simulink model "ppo_position_attitude4drone"  (R2025a)
settings: Solver=ode4  StartTime=0.0  StopTime=50  FixedStep=0.01  RelTol=1e-3
values from neighbouring files (symbols this model uses):
  control_noise = 0.045    [PPO_simulation.mat]    (also in TEST_POS_ATT_PPO.m)
  p_IC = IC(10)    [TEST_POS_ATT_PPO.m]
  phi_IC = IC(7)    [TEST_POS_ATT_PPO.m]
  psi_IC = IC(9)    [TEST_POS_ATT_PPO.m]
  q_IC = IC(11)    [TEST_POS_ATT_PPO.m]
  r_IC = IC(12)    [TEST_POS_ATT_PPO.m]
  state_noise = 0.045    [PPO_simulation.mat]    (also in TEST_POS_ATT_PPO.m)
  theta_IC = IC(8)    [TEST_POS_ATT_PPO.m]
  Ts_Sim = 0.01    [PPO_simulation.mat]    (also in TEST_POS_ATT_PPO.m)
  u_IC = IC(4)    [TEST_POS_ATT_PPO.m]
  v_IC = IC(5)    [TEST_POS_ATT_PPO.m]
  w_IC = IC(6)    [TEST_POS_ATT_PPO.m]
  x_IC = IC(1)    [TEST_POS_ATT_PPO.m]
  y_IC = IC(2)    [TEST_POS_ATT_PPO.m]
  z_IC = IC(3)    [TEST_POS_ATT_PPO.m]
undefined symbols (not defined in the file or in its folder): p_IC2, p_IC3, p_IC4, phi_IC2, phi_IC3, psi_IC2, psi_IC3, q_IC2, q_IC3, r_IC2, r_IC3, saturation_logic, theta_IC2, theta_IC3, u_IC2, u_IC3, v_IC2, v_IC3, w_IC2, w_IC3, wind_logic, x_IC2, x_IC3, y_IC2, y_IC3, z_IC2, z_IC3
libraries: rllib x8
(part 1 of 2)
settings Model: Creator=tn163528  LastModifiedBy=re606359

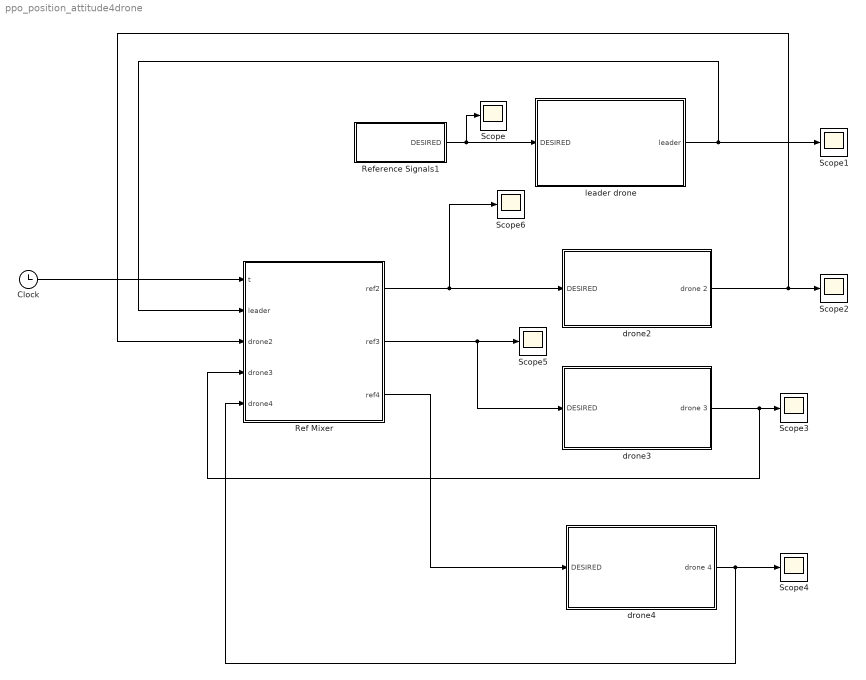
== system ppo_position_attitude4drone ==
  Clock : Clock
  Ref Mixer : MATLAB Function  TreatAsAtomicUnit=on
  Reference Signals1 : Subsystem
  Scope{,1..6} (7 alike) : Scope
      Scope settings: ActiveDisplayYMinimum=-18.329552788512615  ActiveDisplayYMaximum=13.709653230357763  DataLoggingVariableName=ScopeData4
      Scope1 settings: ActiveDisplayYMinimum=-16.8140847666006  ActiveDisplayYMaximum=12.7682316407334  DataLoggingVariableName=ScopeData5
      Scope2 settings: ActiveDisplayYMinimum=-6.2640011047441817  ActiveDisplayYMaximum=4.5374433382914088  DataLoggingVariableName=ScopeData6
      Scope3 settings: ActiveDisplayYMinimum=-16.848247513670785  ActiveDisplayYMaximum=11.660916390407865  DataLoggingVariableName=ScopeData7
      Scope4 settings: ActiveDisplayYMinimum=-16.848247513670785  ActiveDisplayYMaximum=11.660916390407865  DataLoggingVariableName=ScopeData8
      Scope5 settings: ActiveDisplayYMinimum=-2.7528365085187443  ActiveDisplayYMaximum=5.3529951795390245  DataLoggingVariableName=ScopeData9
      Scope6 settings: ActiveDisplayYMinimum=-18.051610011264458  ActiveDisplayYMaximum=3.5641646704603374  DataLoggingVariableName=ScopeData10
  drone2 : Subsystem
  drone3 : Subsystem
  drone4 : Subsystem
  leader drone : Subsystem
  wires:
  Clock/1 -> Ref Mixer/1(t)
  Reference Signals1/1(DESIRED) -> Scope/1, leader drone/1(DESIRED)
  leader drone/1(leader) -> Scope1/1, Ref Mixer/2(leader)
  drone2/1(drone 2) -> Ref Mixer/3(drone2), Scope2/1
  Ref Mixer/1(ref2) -> Scope6/1, drone2/1(DESIRED)
  Ref Mixer/2(ref3) -> drone3/1(DESIRED), Scope5/1
  drone3/1(drone 3) -> Ref Mixer/4(drone3), Scope3/1
  Ref Mixer/3(ref4) -> drone4/1(DESIRED)
  drone4/1(drone 4) -> Ref Mixer/5(drone4), Scope4/1

== system ppo_position_attitude4drone/Reference Signals1 ==
  Clock1 : Clock
  MATLAB Function : MATLAB Function  TreatAsAtomicUnit=on
  Mux : Mux  Inputs=6
  Mux1 : Mux  Inputs=6
  To Workspace : ToWorkspace  VariableName=X_ref  SampleTime=Ts_Sim
  DESIRED : Outport
  wires:
  MATLAB Function/5(z_desir) -> Mux1/3, Mux/5
  MATLAB Function/1(x_desir) -> Mux1/1, Mux/1
  MATLAB Function/6(z_d_desir) -> Mux1/6, Mux/6
  MATLAB Function/2(x_d_desir) -> Mux1/4, Mux/2
  MATLAB Function/3(y_desir) -> Mux1/2, Mux/3
  Mux/1 -> DESIRED/1
  MATLAB Function/4(y_d_desir) -> Mux1/5, Mux/4
  Mux1/1 -> To Workspace/1
  Clock1/1 -> MATLAB Function/1(t)

== system ppo_position_attitude4drone/drone2 ==
  DESIRED : Inport
  Clock : Clock
  Drone_Dynamic1 : Subsystem
  PPO_attitude_controller : Subsystem
  PPO_position_controller : Subsystem
  Scope : Scope  NumInputPorts=3
      settings: ActiveDisplayYMinimum=-0.22794541157782078  ActiveDisplayYMaximum=0.65998090244829655  DataLoggingVariableName=ScopeData2
  Scope1 : Scope
      settings: ActiveDisplayYMinimum=9.7400799288833344  ActiveDisplayYMaximum=10.440050935310733
  System_Solver : MATLAB Function  TreatAsAtomicUnit=on
  drone 2 : Outport
  wires:
  DESIRED/1 -> PPO_position_controller/1(DESIRED)
  PPO_position_controller/3(Uz) -> System_Solver/3(u_z)
  PPO_attitude_controller/1(Taux) -> Scope/3, Drone_Dynamic1/1(tau_x)
  Drone_Dynamic1/1(attitude) -> PPO_attitude_controller/1(actual)  "inner_loop"
  PPO_attitude_controller/2(Tauy) -> Scope/2, Drone_Dynamic1/2(tau_y)
  Drone_Dynamic1/2(position) -> drone 2/1, PPO_position_controller/2(ACTUAL)  "Outer_loop"
  PPO_position_controller/2(Uy) -> System_Solver/2(u_y)
  Clock/1 -> System_Solver/4(t)
  System_Solver/2(theta_desired) -> PPO_attitude_controller/3(theta_desired)
  PPO_attitude_controller/3(Tauz) -> Scope/1, Drone_Dynamic1/3(tau_z)
  System_Solver/1(phi_desired) -> PPO_attitude_controller/2(phi_desired)
  PPO_position_controller/1(Ux) -> System_Solver/1(u_x)
  System_Solver/3(psi_desired) -> PPO_attitude_controller/4(psi_desired)
  System_Solver/4(Ft_desired) -> Drone_Dynamic1/4(F_t), Scope1/1  "F_t"

== system ppo_position_attitude4drone/drone3 ==
  DESIRED : Inport
  Clock : Clock
  Drone_Dynamic1 : Subsystem
  PPO_attitude_controller : Subsystem
  PPO_position_controller : Subsystem
  Scope : Scope  NumInputPorts=3
      settings: ActiveDisplayYMinimum=-0.22794541157782078  ActiveDisplayYMaximum=0.65998090244829655  DataLoggingVariableName=ScopeData2
  Scope1 : Scope
      settings: ActiveDisplayYMinimum=9.7400799288833344  ActiveDisplayYMaximum=10.440050935310733
  System_Solver : MATLAB Function  TreatAsAtomicUnit=on
  drone 3 : Outport
  wires:
  System_Solver/4(Ft_desired) -> Scope1/1, Drone_Dynamic1/4(F_t)  "F_t"
  System_Solver/3(psi_desired) -> PPO_attitude_controller/4(psi_desired)
  PPO_position_controller/1(Ux) -> System_Solver/1(u_x)
  System_Solver/1(phi_desired) -> PPO_attitude_controller/2(phi_desired)
  PPO_attitude_controller/3(Tauz) -> Drone_Dynamic1/3(tau_z), Scope/1
  System_Solver/2(theta_desired) -> PPO_attitude_controller/3(theta_desired)
  Clock/1 -> System_Solver/4(t)
  PPO_position_controller/2(Uy) -> System_Solver/2(u_y)
  Drone_Dynamic1/2(position) -> drone 3/1, PPO_position_controller/2(ACTUAL)  "Outer_loop"
  PPO_attitude_controller/2(Tauy) -> Drone_Dynamic1/2(tau_y), Scope/2
  Drone_Dynamic1/1(attitude) -> PPO_attitude_controller/1(actual)  "inner_loop"
  PPO_attitude_controller/1(Taux) -> Drone_Dynamic1/1(tau_x), Scope/3
  PPO_position_controller/3(Uz) -> System_Solver/3(u_z)
  DESIRED/1 -> PPO_position_controller/1(DESIRED)

== system ppo_position_attitude4drone/drone4 ==
  DESIRED : Inport
  Clock : Clock
  Drone_Dynamic1 : Subsystem
  PPO_attitude_controller : Subsystem
  PPO_position_controller : Subsystem
  Scope : Scope  NumInputPorts=3
      settings: ActiveDisplayYMinimum=-0.22794541157782078  ActiveDisplayYMaximum=0.65998090244829655  DataLoggingVariableName=ScopeData2
  Scope1 : Scope
      settings: ActiveDisplayYMinimum=9.7400799288833344  ActiveDisplayYMaximum=10.440050935310733
  System_Solver : MATLAB Function  TreatAsAtomicUnit=on
  drone 4 : Outport
  wires:
  DESIRED/1 -> PPO_position_controller/1(DESIRED)
  PPO_position_controller/3(Uz) -> System_Solver/3(u_z)
  PPO_attitude_controller/1(Taux) -> Scope/3, Drone_Dynamic1/1(tau_x)
  Drone_Dynamic1/1(attitude) -> PPO_attitude_controller/1(actual)  "inner_loop"
  PPO_attitude_controller/2(Tauy) -> Scope/2, Drone_Dynamic1/2(tau_y)
  Drone_Dynamic1/2(position) -> PPO_position_controller/2(ACTUAL), drone 4/1  "Outer_loop"
  PPO_position_controller/2(Uy) -> System_Solver/2(u_y)
  Clock/1 -> System_Solver/4(t)
  System_Solver/2(theta_desired) -> PPO_attitude_controller/3(theta_desired)
  PPO_attitude_controller/3(Tauz) -> Scope/1, Drone_Dynamic1/3(tau_z)
  System_Solver/1(phi_desired) -> PPO_attitude_controller/2(phi_desired)
  PPO_position_controller/1(Ux) -> System_Solver/1(u_x)
  System_Solver/3(psi_desired) -> PPO_attitude_controller/4(psi_desired)
  System_Solver/4(Ft_desired) -> Drone_Dynamic1/4(F_t), Scope1/1  "F_t"

== system ppo_position_attitude4drone/leader drone ==
  DESIRED : Inport
  Clock : Clock
  Drone_Dynamic1 : Subsystem
  PPO_attitude_controller : Subsystem
  PPO_position_controller : Subsystem
  Scope : Scope  NumInputPorts=3
      settings: ActiveDisplayYMinimum=-0.26589944162275436  ActiveDisplayYMaximum=0.67670267800432526  DataLoggingVariableName=ScopeData12
  Scope1 : Scope
      settings: ActiveDisplayYMinimum=72.877153012049746  ActiveDisplayYMaximum=83.875579825299113  DataLoggingVariableName=ScopeData13
  System_Solver : MATLAB Function  TreatAsAtomicUnit=on
  leader : Outport
  wires:
  System_Solver/4(Ft_desired) -> Scope1/1, Drone_Dynamic1/4(F_t)  "F_t"
  PPO_attitude_controller/1(Taux) -> Drone_Dynamic1/1(tau_x), Scope/3
  System_Solver/1(phi_desired) -> PPO_attitude_controller/2(phi_desired)
  Clock/1 -> System_Solver/4(t)
  DESIRED/1 -> PPO_position_controller/1(DESIRED)
  PPO_position_controller/1(Ux) -> System_Solver/1(u_x)
  System_Solver/2(theta_desired) -> PPO_attitude_controller/3(theta_desired)
  Drone_Dynamic1/1(attitude) -> PPO_attitude_controller/1(actual)  "inner_loop"
  System_Solver/3(psi_desired) -> PPO_attitude_controller/4(psi_desired)
  PPO_position_controller/2(Uy) -> System_Solver/2(u_y)
  Drone_Dynamic1/2(position) -> leader/1, PPO_position_controller/2(ACTUAL)  "Outer_loop"
  PPO_position_controller/3(Uz) -> System_Solver/3(u_z)
  PPO_attitude_controller/2(Tauy) -> Drone_Dynamic1/2(tau_y), Scope/2
  PPO_attitude_controller/3(Tauz) -> Drone_Dynamic1/3(tau_z), Scope/1

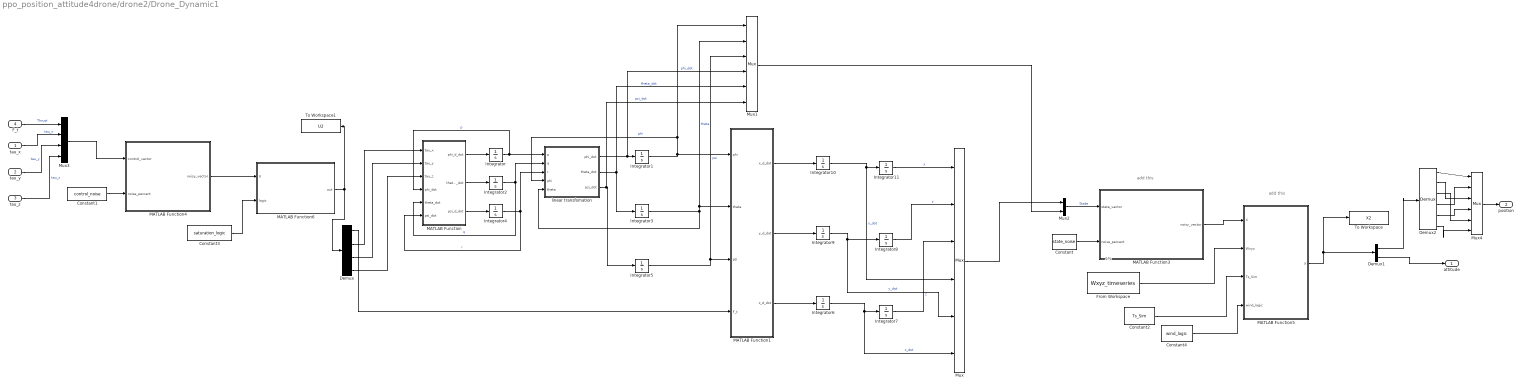
== system ppo_position_attitude4drone/drone2/Drone_Dynamic1 ==
  note: 1%
  note: add this
  note: add this
  tau_x : Inport
  tau_y : Inport  Port=2
  tau_z : Inport  Port=3
  F_t : Inport  Port=4
  Constant : Constant  Value=state_noise  SampleTime=Ts_Sim
  Constant1 : Constant  Value=control_noise
  Constant2 : Constant  Value=Ts_Sim
  Constant3 : Constant  Value=saturation_logic  SampleTime=Ts_Sim
  Constant4 : Constant  Value=wind_logic
  Demux : Demux
  Demux1 : Demux  Outputs=2
  Demux2 : Demux  Outputs=6
  From Workspace : FromWorkspace  VariableName=Wxyz_timeseries  SampleTime=Ts_Sim
  Integrator : Integrator  InitialCondition=p_IC2
  Integrator1 : Integrator  InitialCondition=phi_IC2
  Integrator10 : Integrator  InitialCondition=u_IC2
  Integrator11 : Integrator  InitialCondition=x_IC2
  Integrator2 : Integrator  InitialCondition=q_IC2
  Integrator3 : Integrator  InitialCondition=theta_IC2
  Integrator4 : Integrator  InitialCondition=r_IC2
  Integrator5 : Integrator  InitialCondition=psi_IC2
  Integrator6 : Integrator  InitialCondition=w_IC2
  Integrator7 : Integrator  InitialCondition=z_IC2
  Integrator8 : Integrator  InitialCondition=y_IC2
  Integrator9 : Integrator  InitialCondition=v_IC2
  MATLAB Function : MATLAB Function  TreatAsAtomicUnit=on
  MATLAB Function1 : MATLAB Function  TreatAsAtomicUnit=on
  MATLAB Function3 : MATLAB Function  TreatAsAtomicUnit=on
  MATLAB Function4 : MATLAB Function  TreatAsAtomicUnit=on
  MATLAB Function5 : MATLAB Function  TreatAsAtomicUnit=on
  MATLAB Function6 : MATLAB Function  TreatAsAtomicUnit=on
  Mux : Mux  Inputs=6
  Mux1 : Mux  Inputs=6
  Mux2 : Mux  Inputs=2
  Mux3 : Mux
  Mux4 : Mux  Inputs=6
  To Workspace : ToWorkspace  VariableName=X2  SampleTime=Ts_Sim
  To Workspace1 : ToWorkspace  VariableName=U2  SampleTime=Ts_Sim
  linear transfomation : MATLAB Function  TreatAsAtomicUnit=on
  attitude : Outport
  position : Outport  Port=2
  wires:
  Constant4/1 -> MATLAB Function5/4(wind_logic)
  Mux4/1 -> position/1
  Demux2/6 -> Mux4/6
  Demux2/3 -> Mux4/5
  Demux2/5 -> Mux4/4
  Demux2/2 -> Mux4/3
  Demux2/4 -> Mux4/2
  Demux2/1 -> Mux4/1
  Demux1/1 -> Demux2/1
  Integrator7/1 -> Mux/3  "z"
  Integrator8/1 -> Mux/2  "y"
  Demux/4 -> MATLAB Function/3(tau_z)
  Demux/3 -> MATLAB Function/2(tau_y)
  Demux/2 -> MATLAB Function/1(tau_x)
  Demux/1 -> MATLAB Function1/4(F_t)
  Mux3/1 -> MATLAB Function4/1(control_vector)
  tau_z/1 -> Mux3/4  "tau_z"
  tau_y/1 -> Mux3/3  "tau_y"
  tau_x/1 -> Mux3/2  "tau_x"
  F_t/1 -> Mux3/1  "Thrust"
  Constant1/1 -> MATLAB Function4/2(noise_percent)
  MATLAB Function6/1(out) -> To Workspace1/1, Demux/1
  Constant3/1 -> MATLAB Function6/2(logic)
  MATLAB Function4/1(noisy_vector) -> MATLAB Function6/1(U)
  Mux1/1 -> Mux2/2
  Mux/1 -> Mux2/1
  MATLAB Function5/1(X) -> Demux1/1, To Workspace/1
  Constant2/1 -> MATLAB Function5/3(Ts_Sim)
  From Workspace/1 -> MATLAB Function5/2(Wxyz)
  Demux1/2 -> attitude/1
  MATLAB Function3/1(noisy_vector) -> MATLAB Function5/1("X ")
  Constant/1 -> MATLAB Function3/2(noise_percent)
  Mux2/1 -> MATLAB Function3/1(state_vector)  "State"
  Integrator11/1 -> Mux/1  "x"
  linear transfomation/3(psi_dot) -> Integrator5/1, Mux1/6  "psi_dot"
  linear transfomation/2(theta_dot) -> Integrator3/1, Mux1/5  "theta_dot"
  linear transfomation/1(phi_dot) -> Integrator1/1, Mux1/4  "phi_dot"
  MATLAB Function/2(theta_d_dot) -> Integrator2/1
  MATLAB Function/1(phi_d_dot) -> Integrator/1
  MATLAB Function/3(psi_d_dot) -> Integrator4/1
  Integrator/1 -> linear transfomation/1(p), MATLAB Function/4(phi_dot)  "p"
  Integrator4/1 -> linear transfomation/3(r), MATLAB Function/6(psi_dot)  "r"
  Integrator2/1 -> linear transfomation/2(q), MATLAB Function/5(theta_dot)  "q"
  Integrator6/1 -> Integrator7/1, Mux/6  "z_dot"
  Integrator9/1 -> Integrator8/1, Mux/5  "y_dot"
  Integrator10/1 -> Integrator11/1, Mux/4  "x_dot"
  Integrator5/1 -> MATLAB Function1/3(psi), Mux1/3  "psi"
  Integrator3/1 -> linear transfomation/5(theta), MATLAB Function1/2(theta), Mux1/2  "theta"
  Integrator1/1 -> MATLAB Function1/1(phi), linear transfomation/4(phi), Mux1/1  "phi"
  MATLAB Function1/3(z_d_dot) -> Integrator6/1
  MATLAB Function1/2(y_d_dot) -> Integrator9/1
  MATLAB Function1/1(x_d_dot) -> Integrator10/1

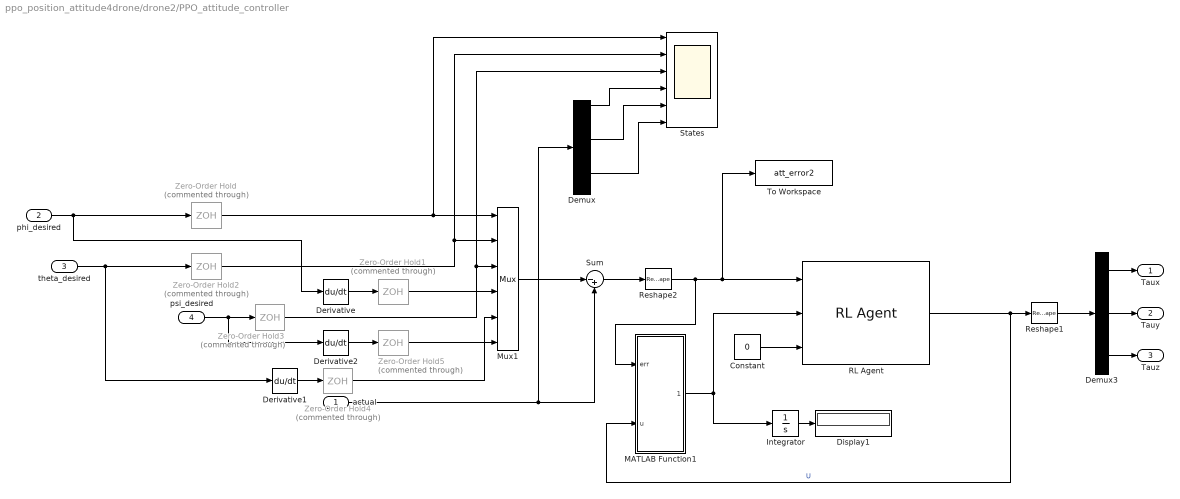
== system ppo_position_attitude4drone/drone2/PPO_attitude_controller ==
  actual : Inport
  phi_desired : Inport  Port=2
  theta_desired : Inport  Port=3
  psi_desired : Inport  Port=4
  Constant : Constant  Value=0
  Demux : Demux  Outputs=6
  Demux3 : Demux  Outputs=3
  Derivative : Derivative
  Derivative1 : Derivative
  Derivative2 : Derivative
  Display1 : Display
  Integrator : Integrator
  MATLAB Function1 : MATLAB Function  TreatAsAtomicUnit=on
  Mux1 : Mux  Inputs=6
  RL Agent : rllib/RL Agent  Agent=agent1  ExternalActionAsInput=off  ProvideLastAction=off  ProvideCumRwd=off  TreatAsDirectFeedthrough=on  UseStrictObservationDataTypes=off
  Reshape1 : Reshape
  Reshape2 : Reshape  OutputDimensionality=Column vector (2-D)
  States : Scope  NumInputPorts=6
      settings: ActiveDisplayYMinimum=-0.042848507934818772  ActiveDisplayYMaximum=0.10576663107375736
  Sum : Sum  Inputs=|-+
  To Workspace : ToWorkspace  VariableName=att_error2  SampleTime=Ts_Sim
  Zero-Order Hold{,1..5} (6 alike) : ZeroOrderHold  Commented=through  SampleTime=.1
  Taux : Outport
  Tauy : Outport  Port=2
  Tauz : Outport  Port=3
  wires:
  Zero-Order Hold5/1 -> Mux1/6
  Zero-Order Hold4/1 -> Mux1/5
  Zero-Order Hold3/1 -> Mux1/3, States/3
  Zero-Order Hold2/1 -> States/2, Mux1/2
  Zero-Order Hold1/1 -> Mux1/4
  Zero-Order Hold/1 -> States/1, Mux1/1
  Derivative2/1 -> Zero-Order Hold5/1
  Derivative1/1 -> Zero-Order Hold4/1
  Derivative/1 -> Zero-Order Hold1/1
  Demux/5 -> States/6
  Demux/3 -> States/5
  Demux/1 -> States/4
  Integrator/1 -> Display1/1
  MATLAB Function1/1(reward) -> Integrator/1, RL Agent/2
  Reshape2/1 -> MATLAB Function1/1(err), RL Agent/1, To Workspace/1
  Sum/1 -> Reshape2/1
  actual/1 -> Sum/2, Demux/1
  Mux1/1 -> Sum/1
  Reshape1/1 -> Demux3/1
  psi_desired/1 -> Zero-Order Hold3/1, Derivative2/1
  theta_desired/1 -> Derivative1/1, Zero-Order Hold2/1
  phi_desired/1 -> Derivative/1, Zero-Order Hold/1
  Demux3/3 -> Tauz/1
  Demux3/2 -> Tauy/1
  Demux3/1 -> Taux/1
  Constant/1 -> RL Agent/3
  RL Agent/1 -> Reshape1/1, MATLAB Function1/2(u)  "U"

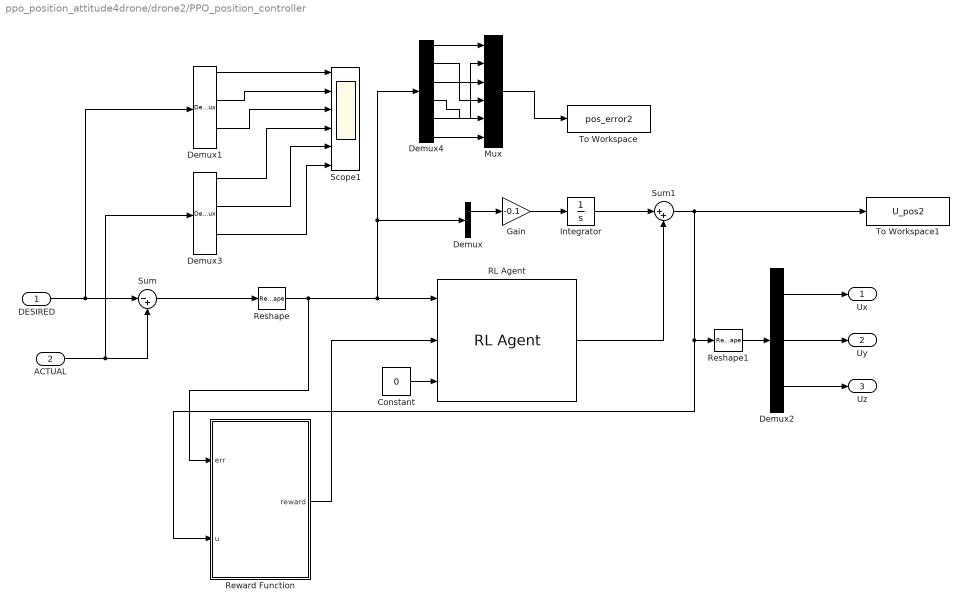
== system ppo_position_attitude4drone/drone2/PPO_position_controller ==
  DESIRED : Inport
  ACTUAL : Inport  Port=2
  Constant : Constant  Value=0
  Demux : Demux  Outputs=2
  Demux1 : Demux  Outputs=6
  Demux2 : Demux  Outputs=3
  Demux3 : Demux  Outputs=6
  Demux4 : Demux  Outputs=6
  Gain : Gain  Gain=-0.1
  Integrator : Integrator
  Mux : Mux  Inputs=6
  RL Agent : rllib/RL Agent  Agent=agent  ExternalActionAsInput=off  ProvideLastAction=off  ProvideCumRwd=off  TreatAsDirectFeedthrough=on  UseStrictObservationDataTypes=off
  Reshape : Reshape  OutputDimensionality=Column vector (2-D)
  Reshape1 : Reshape
  Reward Function : MATLAB Function  TreatAsAtomicUnit=on
  Scope1 : Scope  NumInputPorts=6
      settings: ActiveDisplayYMinimum=-5.046617163465049  ActiveDisplayYMaximum=4.1195544711854284
  Sum : Sum  Inputs=|-+
  Sum1 : Sum  Inputs=|++
  To Workspace : ToWorkspace  VariableName=pos_error2  SampleTime=Ts_Sim
  To Workspace1 : ToWorkspace  VariableName=U_pos2  SampleTime=Ts_Sim
  Ux : Outport
  Uy : Outport  Port=2
  Uz : Outport  Port=3
  wires:
  RL Agent/1 -> Sum1/2
  Demux4/6 -> Mux/6
  Demux4/4 -> Mux/5
  Demux4/5 -> Mux/3
  Demux4/3 -> Mux/2
  Demux4/2 -> Mux/4
  Mux/1 -> To Workspace/1
  Demux4/1 -> Mux/1
  Sum1/1 -> Reshape1/1, Reward Function/2(u), To Workspace1/1
  Integrator/1 -> Sum1/1
  Demux/1 -> Gain/1
  Gain/1 -> Integrator/1
  Demux3/5 -> Scope1/6
  Demux3/3 -> Scope1/5
  Demux3/1 -> Scope1/4
  Demux1/5 -> Scope1/3
  Demux1/3 -> Scope1/2
  Demux1/1 -> Scope1/1
  Constant/1 -> RL Agent/3
  Reshape/1 -> Reward Function/1(err), RL Agent/1, Demux4/1, Demux/1
  Sum/1 -> Reshape/1
  DESIRED/1 -> Sum/1, Demux1/1
  ACTUAL/1 -> Sum/2, Demux3/1
  Reward Function/1(reward) -> RL Agent/2
  Reshape1/1 -> Demux2/1
  Demux2/3 -> Uz/1
  Demux2/2 -> Uy/1
  Demux2/1 -> Ux/1

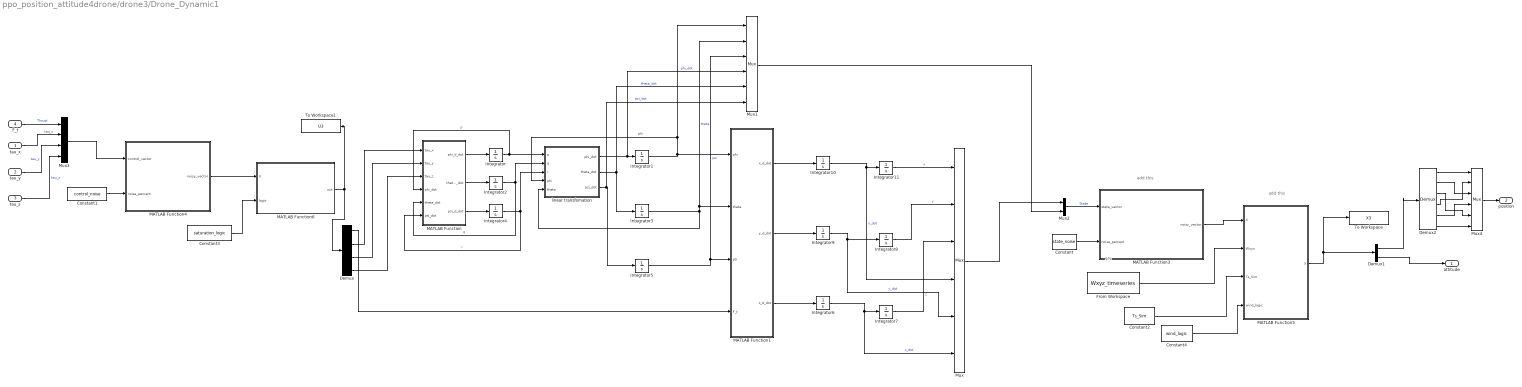
== system ppo_position_attitude4drone/drone3/Drone_Dynamic1 ==
  note: add this
  note: add this
  note: 1%
  tau_x : Inport
  tau_y : Inport  Port=2
  tau_z : Inport  Port=3
  F_t : Inport  Port=4
  Constant : Constant  Value=state_noise  SampleTime=Ts_Sim
  Constant1 : Constant  Value=control_noise
  Constant2 : Constant  Value=Ts_Sim
  Constant3 : Constant  Value=saturation_logic  SampleTime=Ts_Sim
  Constant4 : Constant  Value=wind_logic
  Demux : Demux
  Demux1 : Demux  Outputs=2
  Demux2 : Demux  Outputs=6
  From Workspace : FromWorkspace  VariableName=Wxyz_timeseries  SampleTime=Ts_Sim
  Integrator : Integrator  InitialCondition=p_IC3
  Integrator1 : Integrator  InitialCondition=phi_IC3
  Integrator10 : Integrator  InitialCondition=u_IC3
  Integrator11 : Integrator  InitialCondition=x_IC3
  Integrator2 : Integrator  InitialCondition=q_IC3
  Integrator3 : Integrator  InitialCondition=theta_IC3
  Integrator4 : Integrator  InitialCondition=r_IC3
  Integrator5 : Integrator  InitialCondition=psi_IC3
  Integrator6 : Integrator  InitialCondition=w_IC3
  Integrator7 : Integrator  InitialCondition=z_IC3
  Integrator8 : Integrator  InitialCondition=y_IC3
  Integrator9 : Integrator  InitialCondition=v_IC3
  MATLAB Function : MATLAB Function  TreatAsAtomicUnit=on
  MATLAB Function1 : MATLAB Function  TreatAsAtomicUnit=on
  MATLAB Function3 : MATLAB Function  TreatAsAtomicUnit=on
  MATLAB Function4 : MATLAB Function  TreatAsAtomicUnit=on
  MATLAB Function5 : MATLAB Function  TreatAsAtomicUnit=on
  MATLAB Function6 : MATLAB Function  TreatAsAtomicUnit=on
  Mux : Mux  Inputs=6
  Mux1 : Mux  Inputs=6
  Mux2 : Mux  Inputs=2
  Mux3 : Mux
  Mux4 : Mux  Inputs=6
  To Workspace : ToWorkspace  VariableName=X3  SampleTime=Ts_Sim
  To Workspace1 : ToWorkspace  VariableName=U3  SampleTime=Ts_Sim
  linear transfomation : MATLAB Function  TreatAsAtomicUnit=on
  attitude : Outport
  position : Outport  Port=2
  wires:
  MATLAB Function1/1(x_d_dot) -> Integrator10/1
  MATLAB Function1/2(y_d_dot) -> Integrator9/1
  MATLAB Function1/3(z_d_dot) -> Integrator6/1
  Integrator1/1 -> Mux1/1, linear transfomation/4(phi), MATLAB Function1/1(phi)  "phi"
  Integrator3/1 -> Mux1/2, MATLAB Function1/2(theta), linear transfomation/5(theta)  "theta"
  Integrator5/1 -> Mux1/3, MATLAB Function1/3(psi)  "psi"
  Integrator10/1 -> Mux/4, Integrator11/1  "x_dot"
  Integrator9/1 -> Mux/5, Integrator8/1  "y_dot"
  Integrator6/1 -> Mux/6, Integrator7/1  "z_dot"
  Integrator2/1 -> MATLAB Function/5(theta_dot), linear transfomation/2(q)  "q"
  Integrator4/1 -> MATLAB Function/6(psi_dot), linear transfomation/3(r)  "r"
  Integrator/1 -> MATLAB Function/4(phi_dot), linear transfomation/1(p)  "p"
  MATLAB Function/3(psi_d_dot) -> Integrator4/1
  MATLAB Function/1(phi_d_dot) -> Integrator/1
  MATLAB Function/2(theta_d_dot) -> Integrator2/1
  linear transfomation/1(phi_dot) -> Mux1/4, Integrator1/1  "phi_dot"
  linear transfomation/2(theta_dot) -> Mux1/5, Integrator3/1  "theta_dot"
  linear transfomation/3(psi_dot) -> Mux1/6, Integrator5/1  "psi_dot"
  Integrator11/1 -> Mux/1  "x"
  Mux2/1 -> MATLAB Function3/1(state_vector)  "State"
  Constant/1 -> MATLAB Function3/2(noise_percent)
  MATLAB Function3/1(noisy_vector) -> MATLAB Function5/1("X ")
  Demux1/2 -> attitude/1
  From Workspace/1 -> MATLAB Function5/2(Wxyz)
  Constant2/1 -> MATLAB Function5/3(Ts_Sim)
  MATLAB Function5/1(X) -> To Workspace/1, Demux1/1
  Mux/1 -> Mux2/1
  Mux1/1 -> Mux2/2
  MATLAB Function4/1(noisy_vector) -> MATLAB Function6/1(U)
  Constant3/1 -> MATLAB Function6/2(logic)
  MATLAB Function6/1(out) -> Demux/1, To Workspace1/1
  Constant1/1 -> MATLAB Function4/2(noise_percent)
  F_t/1 -> Mux3/1  "Thrust"
  tau_x/1 -> Mux3/2  "tau_x"
  tau_y/1 -> Mux3/3  "tau_y"
  tau_z/1 -> Mux3/4  "tau_z"
  Mux3/1 -> MATLAB Function4/1(control_vector)
  Demux/1 -> MATLAB Function1/4(F_t)
  Demux/2 -> MATLAB Function/1(tau_x)
  Demux/3 -> MATLAB Function/2(tau_y)
  Demux/4 -> MATLAB Function/3(tau_z)
  Integrator8/1 -> Mux/2  "y"
  Integrator7/1 -> Mux/3  "z"
  Demux1/1 -> Demux2/1
  Demux2/1 -> Mux4/1
  Demux2/4 -> Mux4/2
  Demux2/2 -> Mux4/3
  Demux2/5 -> Mux4/4
  Demux2/3 -> Mux4/5
  Demux2/6 -> Mux4/6
  Mux4/1 -> position/1
  Constant4/1 -> MATLAB Function5/4(wind_logic)

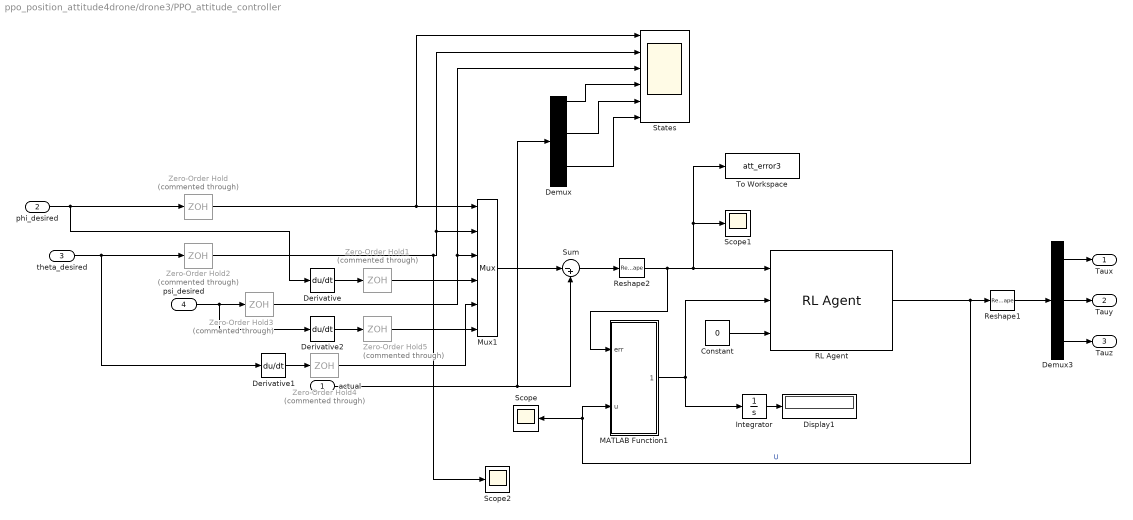
== system ppo_position_attitude4drone/drone3/PPO_attitude_controller ==
  actual : Inport
  phi_desired : Inport  Port=2
  theta_desired : Inport  Port=3
  psi_desired : Inport  Port=4
  Constant : Constant  Value=0
  Demux : Demux  Outputs=6
  Demux3 : Demux  Outputs=3
  Derivative : Derivative
  Derivative1 : Derivative
  Derivative2 : Derivative
  Display1 : Display
  Integrator : Integrator
  MATLAB Function1 : MATLAB Function  TreatAsAtomicUnit=on
  Mux1 : Mux  Inputs=6
  RL Agent : rllib/RL Agent  Agent=agent1  ExternalActionAsInput=off  ProvideLastAction=off  ProvideCumRwd=off  TreatAsDirectFeedthrough=on  UseStrictObservationDataTypes=off
  Reshape1 : Reshape
  Reshape2 : Reshape  OutputDimensionality=Column vector (2-D)
  Scope : Scope
      settings: ActiveDisplayYMinimum=-0.20127  ActiveDisplayYMaximum=0.69251
  Scope1 : Scope
      settings: ActiveDisplayYMinimum=-1  ActiveDisplayYMaximum=1
  Scope2 : Scope
      settings: ActiveDisplayYMinimum=-0.040406254965963853  ActiveDisplayYMaximum=0.036209580605539526  DataLoggingVariableName=ScopeData3
  States : Scope  NumInputPorts=6
      settings: ActiveDisplayYMinimum=-0.042848507934818772  ActiveDisplayYMaximum=0.10576663107375736
  Sum : Sum  Inputs=|-+
  To Workspace : ToWorkspace  VariableName=att_error3  SampleTime=Ts_Sim
  Zero-Order Hold{,1..5} (6 alike) : ZeroOrderHold  Commented=through  SampleTime=.1
  Taux : Outport
  Tauy : Outport  Port=2
  Tauz : Outport  Port=3
  wires:
  RL Agent/1 -> Scope/1, MATLAB Function1/2(u), Reshape1/1  "U"
  Constant/1 -> RL Agent/3
  Demux3/1 -> Taux/1
  Demux3/2 -> Tauy/1
  Demux3/3 -> Tauz/1
  phi_desired/1 -> Zero-Order Hold/1, Derivative/1
  theta_desired/1 -> Zero-Order Hold2/1, Derivative1/1
  psi_desired/1 -> Derivative2/1, Zero-Order Hold3/1
  Reshape1/1 -> Demux3/1
  Mux1/1 -> Sum/1
  actual/1 -> Demux/1, Sum/2
  Sum/1 -> Reshape2/1
  Reshape2/1 -> To Workspace/1, Scope1/1, RL Agent/1, MATLAB Function1/1(err)
  MATLAB Function1/1(reward) -> RL Agent/2, Integrator/1
  Integrator/1 -> Display1/1
  Demux/1 -> States/4
  Demux/3 -> States/5
  Demux/5 -> States/6
  Derivative/1 -> Zero-Order Hold1/1
  Derivative1/1 -> Zero-Order Hold4/1
  Derivative2/1 -> Zero-Order Hold5/1
  Zero-Order Hold/1 -> Mux1/1, States/1
  Zero-Order Hold1/1 -> Mux1/4
  Zero-Order Hold2/1 -> Scope2/1, Mux1/2, States/2
  Zero-Order Hold3/1 -> States/3, Mux1/3
  Zero-Order Hold4/1 -> Mux1/5
  Zero-Order Hold5/1 -> Mux1/6

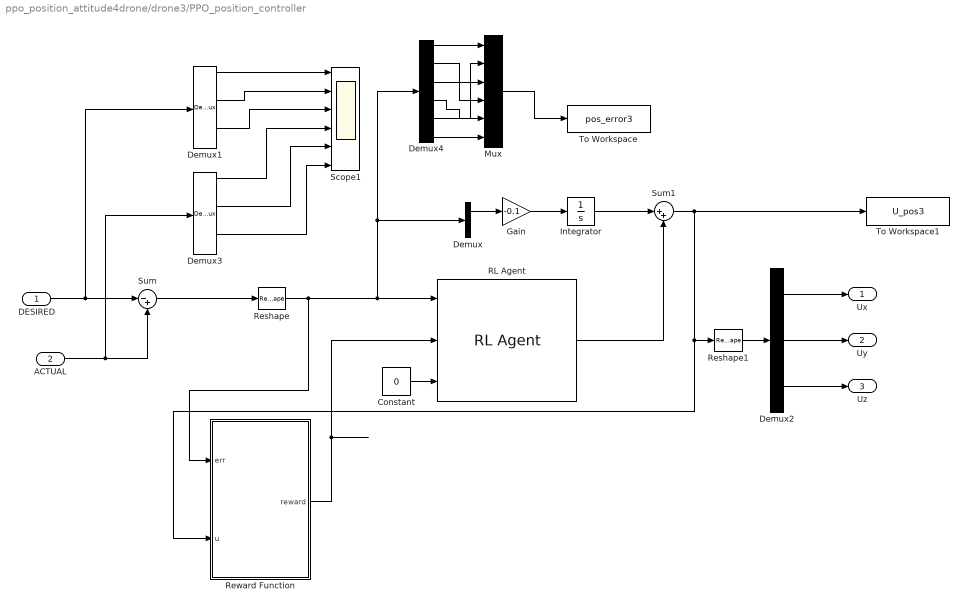
== system ppo_position_attitude4drone/drone3/PPO_position_controller ==
  DESIRED : Inport
  ACTUAL : Inport  Port=2
  Constant : Constant  Value=0
  Demux : Demux  Outputs=2
  Demux1 : Demux  Outputs=6
  Demux2 : Demux  Outputs=3
  Demux3 : Demux  Outputs=6
  Demux4 : Demux  Outputs=6
  Gain : Gain  Gain=-0.1
  Integrator : Integrator
  Mux : Mux  Inputs=6
  RL Agent : rllib/RL Agent  Agent=agent  ExternalActionAsInput=off  ProvideLastAction=off  ProvideCumRwd=off  TreatAsDirectFeedthrough=on  UseStrictObservationDataTypes=off
  Reshape : Reshape  OutputDimensionality=Column vector (2-D)
  Reshape1 : Reshape
  Reward Function : MATLAB Function  TreatAsAtomicUnit=on
  Scope1 : Scope  NumInputPorts=6
      settings: ActiveDisplayYMinimum=-5.046617163465049  ActiveDisplayYMaximum=4.1195544711854284
  Sum : Sum  Inputs=|-+
  Sum1 : Sum  Inputs=|++
  To Workspace : ToWorkspace  VariableName=pos_error3  SampleTime=Ts_Sim
  To Workspace1 : ToWorkspace  VariableName=U_pos3  SampleTime=Ts_Sim
  Ux : Outport
  Uy : Outport  Port=2
  Uz : Outport  Port=3
  wires:
  Demux2/1 -> Ux/1
  Demux2/2 -> Uy/1
  Demux2/3 -> Uz/1
  Reshape1/1 -> Demux2/1
  Reward Function/1(reward) -> RL Agent/2
  ACTUAL/1 -> Demux3/1, Sum/2
  DESIRED/1 -> Demux1/1, Sum/1
  Sum/1 -> Reshape/1
  Reshape/1 -> Demux/1, Demux4/1, RL Agent/1, Reward Function/1(err)
  Constant/1 -> RL Agent/3
  Demux1/1 -> Scope1/1
  Demux1/3 -> Scope1/2
  Demux1/5 -> Scope1/3
  Demux3/1 -> Scope1/4
  Demux3/3 -> Scope1/5
  Demux3/5 -> Scope1/6
  Gain/1 -> Integrator/1
  Demux/1 -> Gain/1
  Integrator/1 -> Sum1/1
  Sum1/1 -> To Workspace1/1, Reward Function/2(u), Reshape1/1
  Demux4/1 -> Mux/1
  Mux/1 -> To Workspace/1
  Demux4/2 -> Mux/4
  Demux4/3 -> Mux/2
  Demux4/5 -> Mux/3
  Demux4/4 -> Mux/5
  Demux4/6 -> Mux/6
  RL Agent/1 -> Sum1/2

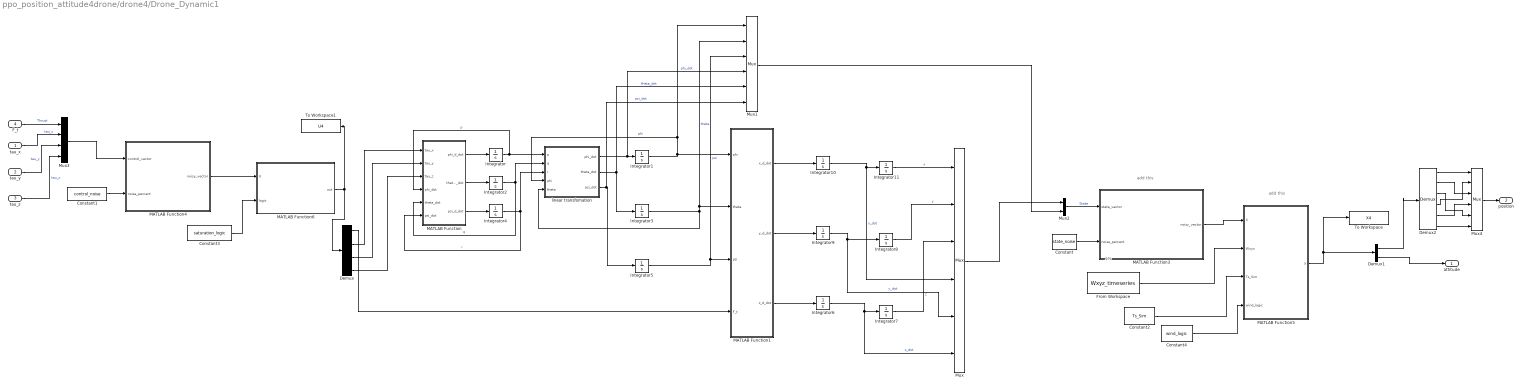
== system ppo_position_attitude4drone/drone4/Drone_Dynamic1 ==
  note: 1%
  note: add this
  note: add this
  tau_x : Inport
  tau_y : Inport  Port=2
  tau_z : Inport  Port=3
  F_t : Inport  Port=4
  Constant : Constant  Value=state_noise  SampleTime=Ts_Sim
  Constant1 : Constant  Value=control_noise
  Constant2 : Constant  Value=Ts_Sim
  Constant3 : Constant  Value=saturation_logic  SampleTime=Ts_Sim
  Constant4 : Constant  Value=wind_logic
  Demux : Demux
  Demux1 : Demux  Outputs=2
  Demux2 : Demux  Outputs=6
  From Workspace : FromWorkspace  VariableName=Wxyz_timeseries  SampleTime=Ts_Sim
  Integrator : Integrator  InitialCondition=p_IC4
  Integrator1 : Integrator  InitialCondition=phi_IC3
  Integrator10 : Integrator  InitialCondition=u_IC3
  Integrator11 : Integrator  InitialCondition=x_IC3
  Integrator2 : Integrator  InitialCondition=q_IC3
  Integrator3 : Integrator  InitialCondition=theta_IC3
  Integrator4 : Integrator  InitialCondition=r_IC3
  Integrator5 : Integrator  InitialCondition=psi_IC3
  Integrator6 : Integrator  InitialCondition=w_IC3
  Integrator7 : Integrator  InitialCondition=z_IC3
  Integrator8 : Integrator  InitialCondition=y_IC3
  Integrator9 : Integrator  InitialCondition=v_IC3
  MATLAB Function : MATLAB Function  TreatAsAtomicUnit=on
  MATLAB Function1 : MATLAB Function  TreatAsAtomicUnit=on
  MATLAB Function3 : MATLAB Function  TreatAsAtomicUnit=on
  MATLAB Function4 : MATLAB Function  TreatAsAtomicUnit=on
  MATLAB Function5 : MATLAB Function  TreatAsAtomicUnit=on
  MATLAB Function6 : MATLAB Function  TreatAsAtomicUnit=on
  Mux : Mux  Inputs=6
  Mux1 : Mux  Inputs=6
  Mux2 : Mux  Inputs=2
  Mux3 : Mux
  Mux4 : Mux  Inputs=6
  To Workspace : ToWorkspace  VariableName=X4  SampleTime=Ts_Sim
  To Workspace1 : ToWorkspace  VariableName=U4  SampleTime=Ts_Sim
  linear transfomation : MATLAB Function  TreatAsAtomicUnit=on
  attitude : Outport
  position : Outport  Port=2
  wires:
  Constant4/1 -> MATLAB Function5/4(wind_logic)
  Mux4/1 -> position/1
  Demux2/6 -> Mux4/6
  Demux2/3 -> Mux4/5
  Demux2/5 -> Mux4/4
  Demux2/2 -> Mux4/3
  Demux2/4 -> Mux4/2
  Demux2/1 -> Mux4/1
  Demux1/1 -> Demux2/1
  Integrator7/1 -> Mux/3  "z"
  Integrator8/1 -> Mux/2  "y"
  Demux/4 -> MATLAB Function/3(tau_z)
  Demux/3 -> MATLAB Function/2(tau_y)
  Demux/2 -> MATLAB Function/1(tau_x)
  Demux/1 -> MATLAB Function1/4(F_t)
  Mux3/1 -> MATLAB Function4/1(control_vector)
  tau_z/1 -> Mux3/4  "tau_z"
  tau_y/1 -> Mux3/3  "tau_y"
  tau_x/1 -> Mux3/2  "tau_x"
  F_t/1 -> Mux3/1  "Thrust"
  Constant1/1 -> MATLAB Function4/2(noise_percent)
  MATLAB Function6/1(out) -> To Workspace1/1, Demux/1
  Constant3/1 -> MATLAB Function6/2(logic)
  MATLAB Function4/1(noisy_vector) -> MATLAB Function6/1(U)
  Mux1/1 -> Mux2/2
  Mux/1 -> Mux2/1
  MATLAB Function5/1(X) -> Demux1/1, To Workspace/1
  Constant2/1 -> MATLAB Function5/3(Ts_Sim)
  From Workspace/1 -> MATLAB Function5/2(Wxyz)
  Demux1/2 -> attitude/1
  MATLAB Function3/1(noisy_vector) -> MATLAB Function5/1("X ")
  Constant/1 -> MATLAB Function3/2(noise_percent)
  Mux2/1 -> MATLAB Function3/1(state_vector)  "State"
  Integrator11/1 -> Mux/1  "x"
  linear transfomation/3(psi_dot) -> Integrator5/1, Mux1/6  "psi_dot"
  linear transfomation/2(theta_dot) -> Integrator3/1, Mux1/5  "theta_dot"
  linear transfomation/1(phi_dot) -> Integrator1/1, Mux1/4  "phi_dot"
  MATLAB Function/2(theta_d_dot) -> Integrator2/1
  MATLAB Function/1(phi_d_dot) -> Integrator/1
  MATLAB Function/3(psi_d_dot) -> Integrator4/1
  Integrator/1 -> linear transfomation/1(p), MATLAB Function/4(phi_dot)  "p"
  Integrator4/1 -> linear transfomation/3(r), MATLAB Function/6(psi_dot)  "r"
  Integrator2/1 -> linear transfomation/2(q), MATLAB Function/5(theta_dot)  "q"
  Integrator6/1 -> Integrator7/1, Mux/6  "z_dot"
  Integrator9/1 -> Integrator8/1, Mux/5  "y_dot"
  Integrator10/1 -> Integrator11/1, Mux/4  "x_dot"
  Integrator5/1 -> MATLAB Function1/3(psi), Mux1/3  "psi"
  Integrator3/1 -> linear transfomation/5(theta), MATLAB Function1/2(theta), Mux1/2  "theta"
  Integrator1/1 -> MATLAB Function1/1(phi), linear transfomation/4(phi), Mux1/1  "phi"
  MATLAB Function1/3(z_d_dot) -> Integrator6/1
  MATLAB Function1/2(y_d_dot) -> Integrator9/1
  MATLAB Function1/1(x_d_dot) -> Integrator10/1

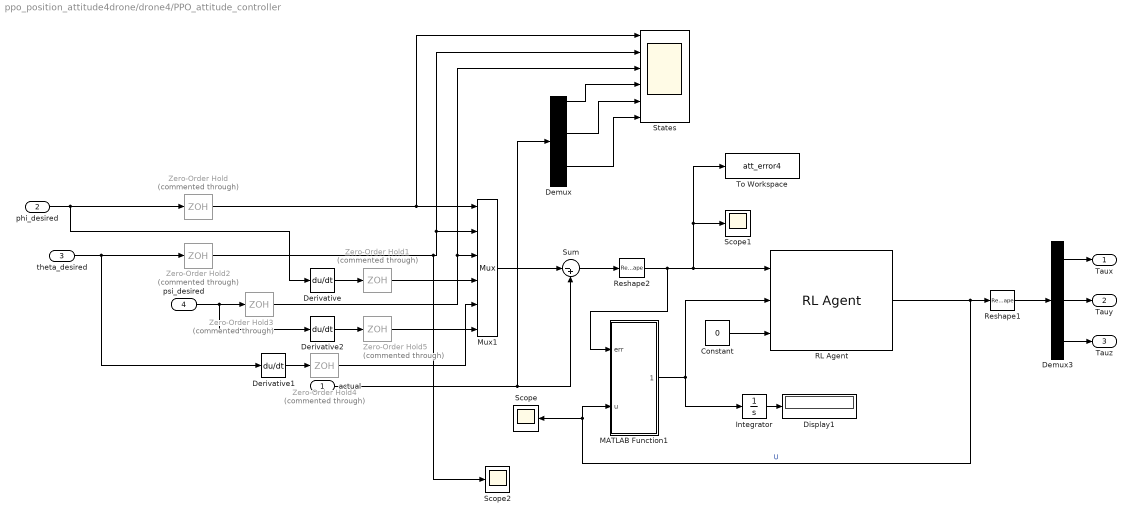
== system ppo_position_attitude4drone/drone4/PPO_attitude_controller ==
  actual : Inport
  phi_desired : Inport  Port=2
  theta_desired : Inport  Port=3
  psi_desired : Inport  Port=4
  Constant : Constant  Value=0
  Demux : Demux  Outputs=6
  Demux3 : Demux  Outputs=3
  Derivative : Derivative
  Derivative1 : Derivative
  Derivative2 : Derivative
  Display1 : Display
  Integrator : Integrator
  MATLAB Function1 : MATLAB Function  TreatAsAtomicUnit=on
  Mux1 : Mux  Inputs=6
  RL Agent : rllib/RL Agent  Agent=agent1  ExternalActionAsInput=off  ProvideLastAction=off  ProvideCumRwd=off  TreatAsDirectFeedthrough=on  UseStrictObservationDataTypes=off
  Reshape1 : Reshape
  Reshape2 : Reshape  OutputDimensionality=Column vector (2-D)
  Scope : Scope
      settings: ActiveDisplayYMinimum=-0.20127  ActiveDisplayYMaximum=0.69251
  Scope1 : Scope
      settings: ActiveDisplayYMinimum=-1  ActiveDisplayYMaximum=1
  Scope2 : Scope
      settings: ActiveDisplayYMinimum=-0.040406254965963853  ActiveDisplayYMaximum=0.036209580605539526  DataLoggingVariableName=ScopeData3
  States : Scope  NumInputPorts=6
      settings: ActiveDisplayYMinimum=-0.042848507934818772  ActiveDisplayYMaximum=0.10576663107375736
  Sum : Sum  Inputs=|-+
  To Workspace : ToWorkspace  VariableName=att_error4  SampleTime=Ts_Sim
  Zero-Order Hold{,1..5} (6 alike) : ZeroOrderHold  Commented=through  SampleTime=.1
  Taux : Outport
  Tauy : Outport  Port=2
  Tauz : Outport  Port=3
  wires:
  Zero-Order Hold5/1 -> Mux1/6
  Zero-Order Hold4/1 -> Mux1/5
  Zero-Order Hold3/1 -> Mux1/3, States/3
  Zero-Order Hold2/1 -> States/2, Mux1/2, Scope2/1
  Zero-Order Hold1/1 -> Mux1/4
  Zero-Order Hold/1 -> States/1, Mux1/1
  Derivative2/1 -> Zero-Order Hold5/1
  Derivative1/1 -> Zero-Order Hold4/1
  Derivative/1 -> Zero-Order Hold1/1
  Demux/5 -> States/6
  Demux/3 -> States/5
  Demux/1 -> States/4
  Integrator/1 -> Display1/1
  MATLAB Function1/1(reward) -> Integrator/1, RL Agent/2
  Reshape2/1 -> MATLAB Function1/1(err), RL Agent/1, Scope1/1, To Workspace/1
  Sum/1 -> Reshape2/1
  actual/1 -> Sum/2, Demux/1
  Mux1/1 -> Sum/1
  Reshape1/1 -> Demux3/1
  psi_desired/1 -> Zero-Order Hold3/1, Derivative2/1
  theta_desired/1 -> Derivative1/1, Zero-Order Hold2/1
  phi_desired/1 -> Derivative/1, Zero-Order Hold/1
  Demux3/3 -> Tauz/1
  Demux3/2 -> Tauy/1
  Demux3/1 -> Taux/1
  Constant/1 -> RL Agent/3
  RL Agent/1 -> Reshape1/1, MATLAB Function1/2(u), Scope/1  "U"

== system ppo_position_attitude4drone/drone4/PPO_position_controller ==
  DESIRED : Inport
  ACTUAL : Inport  Port=2
  Constant : Constant  Value=0
  Demux : Demux  Outputs=2
  Demux1 : Demux  Outputs=6
  Demux2 : Demux  Outputs=3
  Demux3 : Demux  Outputs=6
  Demux4 : Demux  Outputs=6
  Gain : Gain  Gain=-0.1
  Integrator : Integrator
  Mux : Mux  Inputs=6
  RL Agent : rllib/RL Agent  Agent=agent  ExternalActionAsInput=off  ProvideLastAction=off  ProvideCumRwd=off  TreatAsDirectFeedthrough=on  UseStrictObservationDataTypes=off
  Reshape : Reshape  OutputDimensionality=Column vector (2-D)
  Reshape1 : Reshape
  Reward Function : MATLAB Function  TreatAsAtomicUnit=on
  Scope1 : Scope  NumInputPorts=6
      settings: ActiveDisplayYMinimum=-5.046617163465049  ActiveDisplayYMaximum=4.1195544711854284
  Sum : Sum  Inputs=|-+
  Sum1 : Sum  Inputs=|++
  To Workspace : ToWorkspace  VariableName=pos_error4  SampleTime=Ts_Sim
  To Workspace1 : ToWorkspace  VariableName=U_pos4  SampleTime=Ts_Sim
  Ux : Outport
  Uy : Outport  Port=2
  Uz : Outport  Port=3
  wires:
  RL Agent/1 -> Sum1/2
  Demux4/6 -> Mux/6
  Demux4/4 -> Mux/5
  Demux4/5 -> Mux/3
  Demux4/3 -> Mux/2
  Demux4/2 -> Mux/4
  Mux/1 -> To Workspace/1
  Demux4/1 -> Mux/1
  Sum1/1 -> Reshape1/1, Reward Function/2(u), To Workspace1/1
  Integrator/1 -> Sum1/1
  Demux/1 -> Gain/1
  Gain/1 -> Integrator/1
  Demux3/5 -> Scope1/6
  Demux3/3 -> Scope1/5
  Demux3/1 -> Scope1/4
  Demux1/5 -> Scope1/3
  Demux1/3 -> Scope1/2
  Demux1/1 -> Scope1/1
  Constant/1 -> RL Agent/3
  Reshape/1 -> Reward Function/1(err), RL Agent/1, Demux4/1, Demux/1
  Sum/1 -> Reshape/1
  DESIRED/1 -> Sum/1, Demux1/1
  ACTUAL/1 -> Sum/2, Demux3/1
  Reward Function/1(reward) -> RL Agent/2
  Reshape1/1 -> Demux2/1
  Demux2/3 -> Uz/1
  Demux2/2 -> Uy/1
  Demux2/1 -> Ux/1

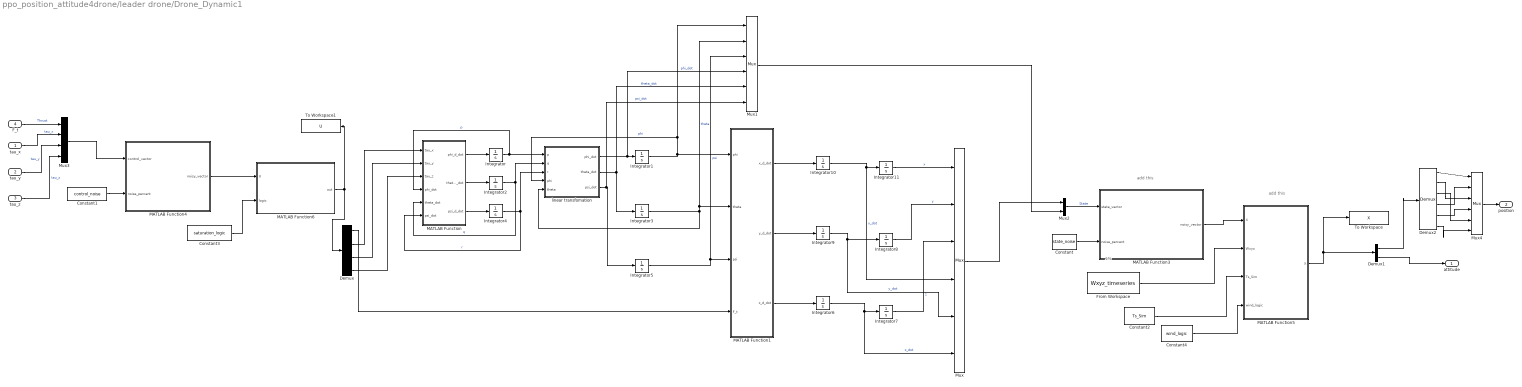
== system ppo_position_attitude4drone/leader drone/Drone_Dynamic1 ==
  note: add this
  note: add this
  note: 1%
  tau_x : Inport
  tau_y : Inport  Port=2
  tau_z : Inport  Port=3
  F_t : Inport  Port=4
  Constant : Constant  Value=state_noise  SampleTime=Ts_Sim
  Constant1 : Constant  Value=control_noise
  Constant2 : Constant  Value=Ts_Sim
  Constant3 : Constant  Value=saturation_logic  SampleTime=Ts_Sim
  Constant4 : Constant  Value=wind_logic
  Demux : Demux
  Demux1 : Demux  Outputs=2
  Demux2 : Demux  Outputs=6
  From Workspace : FromWorkspace  VariableName=Wxyz_timeseries  SampleTime=Ts_Sim
  Integrator : Integrator  InitialCondition=p_IC
  Integrator1 : Integrator  InitialCondition=phi_IC
  Integrator10 : Integrator  InitialCondition=u_IC
  Integrator11 : Integrator  InitialCondition=x_IC
  Integrator2 : Integrator  InitialCondition=q_IC
  Integrator3 : Integrator  InitialCondition=theta_IC
  Integrator4 : Integrator  InitialCondition=r_IC
  Integrator5 : Integrator  InitialCondition=psi_IC
  Integrator6 : Integrator  InitialCondition=w_IC
  Integrator7 : Integrator  InitialCondition=z_IC
  Integrator8 : Integrator  InitialCondition=y_IC
  Integrator9 : Integrator  InitialCondition=v_IC
  MATLAB Function : MATLAB Function  TreatAsAtomicUnit=on
  MATLAB Function1 : MATLAB Function  TreatAsAtomicUnit=on
  MATLAB Function3 : MATLAB Function  TreatAsAtomicUnit=on
  MATLAB Function4 : MATLAB Function  TreatAsAtomicUnit=on
  MATLAB Function5 : MATLAB Function  TreatAsAtomicUnit=on
  MATLAB Function6 : MATLAB Function  TreatAsAtomicUnit=on
  Mux : Mux  Inputs=6
  Mux1 : Mux  Inputs=6
  Mux2 : Mux  Inputs=2
  Mux3 : Mux
  Mux4 : Mux  Inputs=6
  To Workspace : ToWorkspace  VariableName=X  SampleTime=Ts_Sim
  To Workspace1 : ToWorkspace  VariableName=U  SampleTime=Ts_Sim
  linear transfomation : MATLAB Function  TreatAsAtomicUnit=on
  attitude : Outport
  position : Outport  Port=2
  wires:
  MATLAB Function1/1(x_d_dot) -> Integrator10/1
  MATLAB Function1/2(y_d_dot) -> Integrator9/1
  MATLAB Function1/3(z_d_dot) -> Integrator6/1
  Integrator1/1 -> Mux1/1, linear transfomation/4(phi), MATLAB Function1/1(phi)  "phi"
  Integrator3/1 -> Mux1/2, MATLAB Function1/2(theta), linear transfomation/5(theta)  "theta"
  Integrator5/1 -> Mux1/3, MATLAB Function1/3(psi)  "psi"
  Integrator10/1 -> Mux/4, Integrator11/1  "x_dot"
  Integrator9/1 -> Mux/5, Integrator8/1  "y_dot"
  Integrator6/1 -> Mux/6, Integrator7/1  "z_dot"
  Integrator2/1 -> MATLAB Function/5(theta_dot), linear transfomation/2(q)  "q"
  Integrator4/1 -> MATLAB Function/6(psi_dot), linear transfomation/3(r)  "r"
  Integrator/1 -> MATLAB Function/4(phi_dot), linear transfomation/1(p)  "p"
  MATLAB Function/3(psi_d_dot) -> Integrator4/1
  MATLAB Function/1(phi_d_dot) -> Integrator/1
  MATLAB Function/2(theta_d_dot) -> Integrator2/1
  linear transfomation/1(phi_dot) -> Mux1/4, Integrator1/1  "phi_dot"
  linear transfomation/2(theta_dot) -> Mux1/5, Integrator3/1  "theta_dot"
  linear transfomation/3(psi_dot) -> Mux1/6, Integrator5/1  "psi_dot"
  Integrator11/1 -> Mux/1  "x"
  Mux2/1 -> MATLAB Function3/1(state_vector)  "State"
  Constant/1 -> MATLAB Function3/2(noise_percent)
  MATLAB Function3/1(noisy_vector) -> MATLAB Function5/1("X ")
  Demux1/2 -> attitude/1
  From Workspace/1 -> MATLAB Function5/2(Wxyz)
  Constant2/1 -> MATLAB Function5/3(Ts_Sim)
  MATLAB Function5/1(X) -> To Workspace/1, Demux1/1
  Mux/1 -> Mux2/1
  Mux1/1 -> Mux2/2
  MATLAB Function4/1(noisy_vector) -> MATLAB Function6/1(U)
  Constant3/1 -> MATLAB Function6/2(logic)
  MATLAB Function6/1(out) -> Demux/1, To Workspace1/1
  Constant1/1 -> MATLAB Function4/2(noise_percent)
  F_t/1 -> Mux3/1  "Thrust"
  tau_x/1 -> Mux3/2  "tau_x"
  tau_y/1 -> Mux3/3  "tau_y"
  tau_z/1 -> Mux3/4  "tau_z"
  Mux3/1 -> MATLAB Function4/1(control_vector)
  Demux/1 -> MATLAB Function1/4(F_t)
  Demux/2 -> MATLAB Function/1(tau_x)
  Demux/3 -> MATLAB Function/2(tau_y)
  Demux/4 -> MATLAB Function/3(tau_z)
  Integrator8/1 -> Mux/2  "y"
  Integrator7/1 -> Mux/3  "z"
  Demux1/1 -> Demux2/1
  Demux2/1 -> Mux4/1
  Demux2/4 -> Mux4/2
  Demux2/2 -> Mux4/3
  Demux2/5 -> Mux4/4
  Demux2/3 -> Mux4/5
  Demux2/6 -> Mux4/6
  Mux4/1 -> position/1
  Constant4/1 -> MATLAB Function5/4(wind_logic)

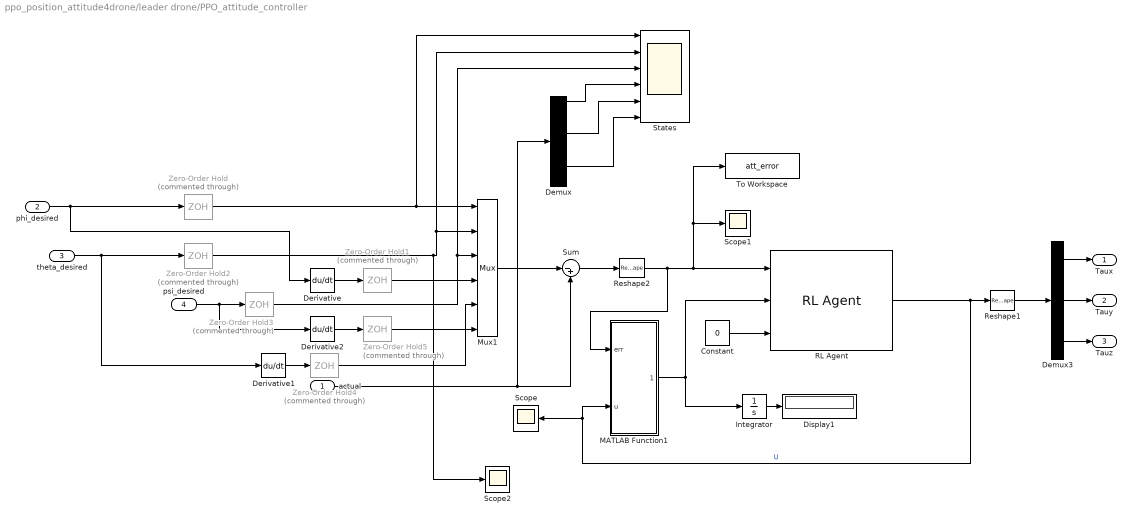
== system ppo_position_attitude4drone/leader drone/PPO_attitude_controller ==
  actual : Inport
  phi_desired : Inport  Port=2
  theta_desired : Inport  Port=3
  psi_desired : Inport  Port=4
  Constant : Constant  Value=0
  Demux : Demux  Outputs=6
  Demux3 : Demux  Outputs=3
  Derivative : Derivative
  Derivative1 : Derivative
  Derivative2 : Derivative
  Display1 : Display
  Integrator : Integrator
  MATLAB Function1 : MATLAB Function  TreatAsAtomicUnit=on
  Mux1 : Mux  Inputs=6
  RL Agent : rllib/RL Agent  Agent=agent1  ExternalActionAsInput=off  ProvideLastAction=off  ProvideCumRwd=off  TreatAsDirectFeedthrough=on  UseStrictObservationDataTypes=off
  Reshape1 : Reshape
  Reshape2 : Reshape  OutputDimensionality=Column vector (2-D)
  Scope : Scope
      settings: ActiveDisplayYMinimum=-0.20127  ActiveDisplayYMaximum=0.69251
  Scope1 : Scope
      settings: ActiveDisplayYMinimum=-1  ActiveDisplayYMaximum=1
  Scope2 : Scope
      settings: ActiveDisplayYMinimum=-0.040406254965963853  ActiveDisplayYMaximum=0.036209580605539526  DataLoggingVariableName=ScopeData3
  States : Scope  NumInputPorts=6
      settings: ActiveDisplayYMinimum=-0.042848507934818772  ActiveDisplayYMaximum=0.10576663107375736
  Sum : Sum  Inputs=|-+
  To Workspace : ToWorkspace  VariableName=att_error  SampleTime=Ts_Sim
  Zero-Order Hold{,1..5} (6 alike) : ZeroOrderHold  Commented=through  SampleTime=.1
  Taux : Outport
  Tauy : Outport  Port=2
  Tauz : Outport  Port=3
  wires:
  RL Agent/1 -> Scope/1, MATLAB Function1/2(u), Reshape1/1  "U"
  Constant/1 -> RL Agent/3
  Demux3/1 -> Taux/1
  Demux3/2 -> Tauy/1
  Demux3/3 -> Tauz/1
  phi_desired/1 -> Zero-Order Hold/1, Derivative/1
  theta_desired/1 -> Zero-Order Hold2/1, Derivative1/1
  psi_desired/1 -> Derivative2/1, Zero-Order Hold3/1
  Reshape1/1 -> Demux3/1
  Mux1/1 -> Sum/1
  actual/1 -> Demux/1, Sum/2
  Sum/1 -> Reshape2/1
  Reshape2/1 -> To Workspace/1, Scope1/1, RL Agent/1, MATLAB Function1/1(err)
  MATLAB Function1/1(reward) -> RL Agent/2, Integrator/1
  Integrator/1 -> Display1/1
  Demux/1 -> States/4
  Demux/3 -> States/5
  Demux/5 -> States/6
  Derivative/1 -> Zero-Order Hold1/1
  Derivative1/1 -> Zero-Order Hold4/1
  Derivative2/1 -> Zero-Order Hold5/1
  Zero-Order Hold/1 -> Mux1/1, States/1
  Zero-Order Hold1/1 -> Mux1/4
  Zero-Order Hold2/1 -> Scope2/1, Mux1/2, States/2
  Zero-Order Hold3/1 -> States/3, Mux1/3
  Zero-Order Hold4/1 -> Mux1/5
  Zero-Order Hold5/1 -> Mux1/6

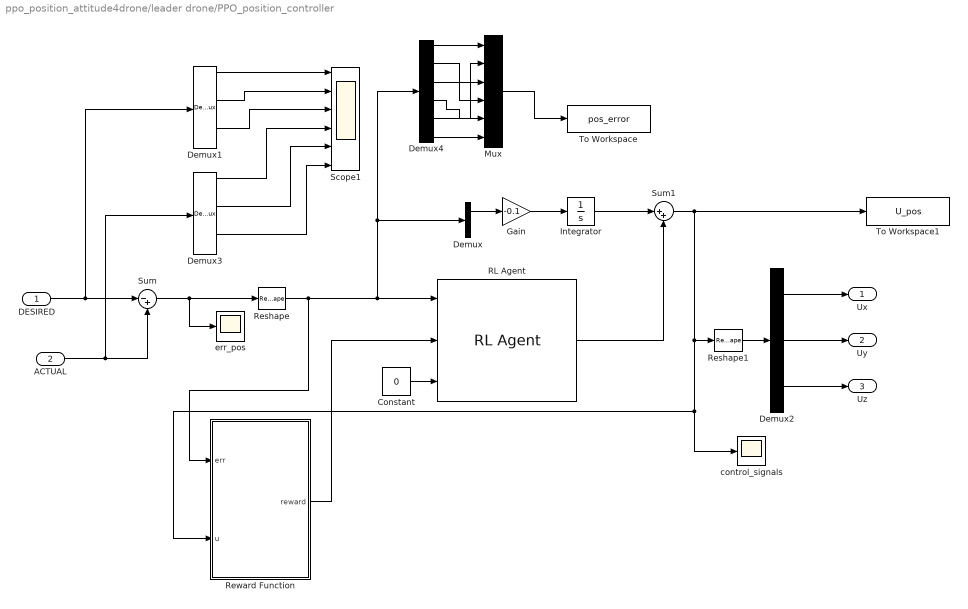
== system ppo_position_attitude4drone/leader drone/PPO_position_controller ==
  DESIRED : Inport
  ACTUAL : Inport  Port=2
  Constant : Constant  Value=0
  Demux : Demux  Outputs=2
  Demux1 : Demux  Outputs=6
  Demux2 : Demux  Outputs=3
  Demux3 : Demux  Outputs=6
  Demux4 : Demux  Outputs=6
  Gain : Gain  Gain=-0.1
  Integrator : Integrator
  Mux : Mux  Inputs=6
  RL Agent : rllib/RL Agent  Agent=agent  ExternalActionAsInput=off  ProvideLastAction=off  ProvideCumRwd=off  TreatAsDirectFeedthrough=on  UseStrictObservationDataTypes=off
  Reshape : Reshape  OutputDimensionality=Column vector (2-D)
  Reshape1 : Reshape
  Reward Function : MATLAB Function  TreatAsAtomicUnit=on
  Scope1 : Scope  NumInputPorts=6
      settings: ActiveDisplayYMinimum=-5.046617163465049  ActiveDisplayYMaximum=4.1195544711854284
  Sum : Sum  Inputs=|-+
  Sum1 : Sum  Inputs=|++
  To Workspace : ToWorkspace  VariableName=pos_error  SampleTime=Ts_Sim
  To Workspace1 : ToWorkspace  VariableName=U_pos  SampleTime=Ts_Sim
  control_signals : Scope
      settings: ActiveDisplayYMinimum=-0.47076  ActiveDisplayYMaximum=0.3367  DataLoggingVariableName=control_signal
  err_pos : Scope
      settings: ActiveDisplayYMinimum=-2.9375  ActiveDisplayYMaximum=1.4375  DataLoggingVariableName=control_signal1
  Ux : Outport
  Uy : Outport  Port=2
  Uz : Outport  Port=3
  wires:
  Demux2/1 -> Ux/1
  Demux2/2 -> Uy/1
  Demux2/3 -> Uz/1
  Reshape1/1 -> Demux2/1
  Reward Function/1(reward) -> RL Agent/2
  ACTUAL/1 -> Demux3/1, Sum/2
  DESIRED/1 -> Demux1/1, Sum/1
  Sum/1 -> Reshape/1, err_pos/1
  Reshape/1 -> Demux/1, Demux4/1, RL Agent/1, Reward Function/1(err)
  Constant/1 -> RL Agent/3
  Demux1/1 -> Scope1/1
  Demux1/3 -> Scope1/2
  Demux1/5 -> Scope1/3
  Demux3/1 -> Scope1/4
  Demux3/3 -> Scope1/5
  Demux3/5 -> Scope1/6
  Gain/1 -> Integrator/1
  Demux/1 -> Gain/1
  Integrator/1 -> Sum1/1
  Sum1/1 -> To Workspace1/1, control_signals/1, Reward Function/2(u), Reshape1/1
  Demux4/1 -> Mux/1
  Mux/1 -> To Workspace/1
  Demux4/2 -> Mux/4
  Demux4/3 -> Mux/2
  Demux4/5 -> Mux/3
  Demux4/4 -> Mux/5
  Demux4/6 -> Mux/6
  RL Agent/1 -> Sum1/2

== matlab function ppo_position_attitude4drone/leader drone/Drone_Dynamic1/linear transfomation ==
  data: p input; q input; r input; phi_dot output; phi input; theta input; theta_dot output; psi_dot output
function [phi_dot, theta_dot, psi_dot] = fcn(p,q,r, phi,theta)

    phi_dot   = p + (q*sin(phi)*tan(theta)) + (r*cos(phi)*tan(theta));
    theta_dot = (q*cos(phi)) - (r*sin(phi));
    psi_dot   = (q*sin(phi)/cos(theta)) + (r*cos(phi)/cos(theta));

end



    % if theta == deg2rad(90) || theta == deg2rad(-90)
    %    theta = sign(theta)*deg2rad(89.9); 
    % end

% 89.9 value is fixed. 
% if change to 89.99, phi_dot and psi_dot value will explode.

== matlab function ppo_position_attitude4drone/leader drone/Drone_Dynamic1/MATLAB Function4 ==
  settings: updateMethod=DISCRETE
  data: control_vector input; noisy_vector output; noise_percent input
function noisy_vector = add_control_noise(control_vector, noise_percent)

    L = 0.2;
    % drag = 0.02; % (drag coef)
    max_Ft = 2*9.81;
    Tmax = max_Ft/4;
    Max_torque = Tmax*L*2;
    actuator_uncert = [0.1*max_Ft, 0.01*Max_torque, 0.01*Max_torque, 0.02*Max_torque]';
    
    noise = (noise_percent) * actuator_uncert .* randn(size(control_vector)); % noise_percent 1 2 3 4 5
    noisy_vector = control_vector + noise;
    
end

== matlab function ppo_position_attitude4drone/leader drone/Drone_Dynamic1/MATLAB Function6 ==
  data: U input; out output; logic input
% saturation function
function out = saturate_controls(U, logic)

    if logic == 1

        ft = U(1);
        torques = [U(2); U(3); U(4)];
        m = 1;
        g = 9.81;
        L = 0.2;
        drag = 0.02; % (drag coef)
        max_Ft = 2*m*g;
        Tmin = 0;
        Tmax = max_Ft/4;
        max_torque = Tmax*L*2;
        max_yaw_torque = 0.7*max_torque;

        % saturate the torques to the max torque the drone can produce
        for p = 1:2 % sat the first 2
            if torques(p) > max_torque
                torques(p) = max_torque;
            elseif torques(p) < -max_torque
                torques(p) = -max_torque;
            end
        end
        if torques(3) > max_yaw_torque
            torques(3) = max_yaw_torque;
        elseif torques(3) < -max_yaw_torque
            torques(3) = -max_yaw_torque;
        end
        % solve for the thrust of each motor given those torques
        T1 = (ft - torques(1)/(2*L) - torques(2)/(2*L) + torques(3)/(4*drag)) / 4;
        T2 = (ft - torques(1)/(2*L) + torques(2)/(2*L) + torques(3)/(4*drag)) / 4;
        T3 = (ft + torques(1)/(2*L) - torques(2)/(2*L) - torques(3)/(4*drag)) / 4;
        T4 = (ft + torques(1)/(2*L) + torques(2)/(2*L) - torques(3)/(4*drag)) / 4;
        each_motor_thrust = [T1;T2;T3;T4];

        % saturate each motor thrust to its bounded values
        for j = 1:4
            if each_motor_thrust(j) > Tmax
                each_motor_thrust(j) = Tmax;
            elseif each_motor_thrust(j) < Tmin
                each_motor_thrust(j) = Tmin;
            end
        end

        ft = sum(each_motor_thrust);

        if ft>max_Ft
            ft = max_Ft;
        elseif ft<0
            ft = 0;
        end

        out = [ft; torques];

    else
    
        out = U;
    
    end


end

== matlab function ppo_position_attitude4drone/drone2/Drone_Dynamic1/MATLAB Function ==
  data: tau_x input; tau_y input; tau_z input; phi_d_dot output; theta_d_dot output; psi_d_dot output; phi_dot input; theta_dot input; psi_dot input
function [phi_d_dot, theta_d_dot, psi_d_dot] = fcn(tau_x, tau_y, tau_z, phi_dot, theta_dot, psi_dot)
    I_x = 0.3; I_y = 0.4; I_z = 0.5;
    phi_d_dot = (((I_y - I_z)/I_x) * theta_dot * psi_dot) + (tau_x/I_x);
    theta_d_dot = (((I_z - I_x)/I_y) * phi_dot * psi_dot) + (tau_y/I_y);
    psi_d_dot = (((I_x - I_y)/I_z) * phi_dot * psi_dot) + (tau_z/I_z);
end

== matlab function ppo_position_attitude4drone/drone2/Drone_Dynamic1/MATLAB Function1 ==
  data: phi input; x_d_dot output; theta input; psi input; F_t input; y_d_dot output; z_d_dot output
function [x_d_dot, y_d_dot, z_d_dot] = fcn(phi, theta, psi, F_t)
    m = 1; %1kg
    g = 9.81;
    x_d_dot= -(F_t/m) * (sin(phi)*sin(psi) + cos(phi)*cos(psi)*sin(theta));
    y_d_dot= -(F_t/m) * (cos(phi)*sin(psi)*sin(theta) - cos(psi)*sin(phi));
    z_d_dot= g-(F_t/m) * (cos(phi) * cos(theta));
end

== matlab function ppo_position_attitude4drone/drone2/Drone_Dynamic1/MATLAB Function3 ==
  settings: updateMethod=DISCRETE
  data: state_vector input; noisy_vector output; noise_percent input
function noisy_vector = add_state_noise(state_vector,noise_percent)

    sensor_uncert = [0.02, 0.02, 0.05, 0.05, 0.05, 0.05, 0.15, 0.15, 0.5, 0.005, 0.005, 0.005]';
  
    noise = (noise_percent) * sensor_uncert .* randn(size(state_vector)); % 0.01 usually add noise_percent 1 2 3 4 5
    noisy_vector = state_vector + noise;

end

== matlab function ppo_position_attitude4drone/drone2/Drone_Dynamic1/MATLAB Function4 ==
  settings: updateMethod=DISCRETE
  data: control_vector input; noisy_vector output; noise_percent input
function noisy_vector = add_control_noise(control_vector, noise_percent)

    L = 0.2;
    % drag = 0.02; % (drag coef)
    max_Ft = 2*9.81;
    Tmax = max_Ft/4;
    Max_torque = Tmax*L*2;
    actuator_uncert = [0.1*max_Ft, 0.01*Max_torque, 0.01*Max_torque, 0.02*Max_torque]';
    
    noise = (noise_percent) * actuator_uncert .* randn(size(control_vector)); % noise_percent 1 2 3 4 5
    noisy_vector = control_vector + noise;
    
end
